simulink model "SecRwRtStBkReclnCtrl"  (R2024b)
settings: Solver=FixedStepDiscrete  StartTime=0.0  StopTime=10.0  FixedStep=0.01  RelTol=1e-3
undefined symbols (not defined in the file or in its folder): KeSMSuMdMotFinshdTm_Val, KeSMSuMdRetryTm1_Val, KeSMSuModeReqDurgTm_Val
libraries: StCtrlLibBkRecln x1
settings Model: Creator=sn2xws  LastModifiedBy=sn55gm
settings SolverCC: AlgebraicLoopSolver=TrustRegion
settings DataIOCC: SaveFormat=StructureWithTime  ReturnWorkspaceOutputs=off
settings OptimizationCC: DefaultParameterBehavior=Inlined  EnhancedBackFolding=on  PassReuseOutputArgsAs=Individual arguments  ZeroExternalMemoryAtStartup=off  ZeroInternalMemoryAtStartup=off  OptimizeBlockOrder=speed  DifferentSizesBufferReuse=on  OptimizationCustomize=off  EfficientTunableParamExpr=on
settings DebuggingCC: ParameterTunabilityLossMsg=error  UnconnectedInputMsg=warning  UnconnectedOutputMsg=warning  UnconnectedLineMsg=warning  ArithmeticOperatorsInVariantConditions=warning
settings ModelReferenceCC: EnableRefExpFcnMdlSchedulingChecks=on  ModelReferenceNumInstancesAllowed=Single
settings SFSimCC: MATLABDynamicMemAlloc=off  CustomCodeUndefinedFunction=UseInterfaceOnly
settings RTWCC: Description=AUTOSAR  SystemTargetFile=autosar.tlc  GenCodeOnly=on  TemplateMakefile=ert_default_tmf  GenerateReport=on  IncludeHyperlinkInReport=on  LaunchReport=on  DataTypeReplacement=CDataTypesFixedWidth  GenerateTraceInfo=on  GenerateTraceReport=on  GenerateTraceReportSl=on  GenerateTraceReportSf=on  GenerateTraceReportEml=on  GPUComputeCapability=3.5
settings CodeAppCC: ForceParamTrailComments=on  IgnoreCustomStorageClasses=off  OperatorAnnotations=on  SimulinkDataObjDesc=on  SFDataObjDesc=on  InsertBlockDesc=on
settings STFCustomTargetCC: TargetLangStandard=C99 (ISO)  MultiwordLength=256  ParMdlRefBuildCompliant=on  CompOptLevelCompliant=on  IncludeMdlTerminateFcn=off  CombineOutputUpdateFcns=on  SuppressErrorStatus=on  ERTCustomFileBanners=on  SupportNonFinite=off  SupportComplex=off  SupportContinuousTime=off  SupportNonInlinedSFcns=off  RemoveResetFunc=on  MATLABClassNameForMDSCustomization=Simulink.SoftwareTarget.ERTCustomization  AutosarCompliant=on  UseToolchainInfoCompliant=on  LookupTableObjectStructAxisOrder=2,1,3,4,...  LUTObjectStructOrderEvenSpacing=Size,Table,Breakpoints  SystemTargetFile=autosar.tlc
settings ERTTargetCC: TargetLangStandard=C99 (ISO)  ConcurrentExecutionCompliant=off  IncludeMdlTerminateFcn=off  SuppressErrorStatus=on  SupportNonFinite=off  SupportComplex=off  ModelStepFunctionPrototypeControlCompliant=off  CPPClassGenCompliant=off  AutosarCompliant=on  LookupTableObjectStructAxisOrder=2,1,3,4,...  LUTObjectStructOrderEvenSpacing=Size,Table,Breakpoints  ERTCustomFileTemplate=example_file_process.tlc  ERTFilePackagingFormat=Compact  BooleanTrueId=TRUE  BooleanFalseId=FALSE  DynamicArrayContainerType=coder::array

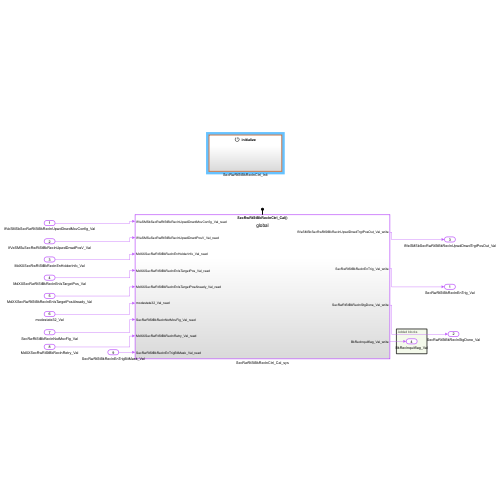
[thumbnail: Simulink's stored preview of the top-level diagram]
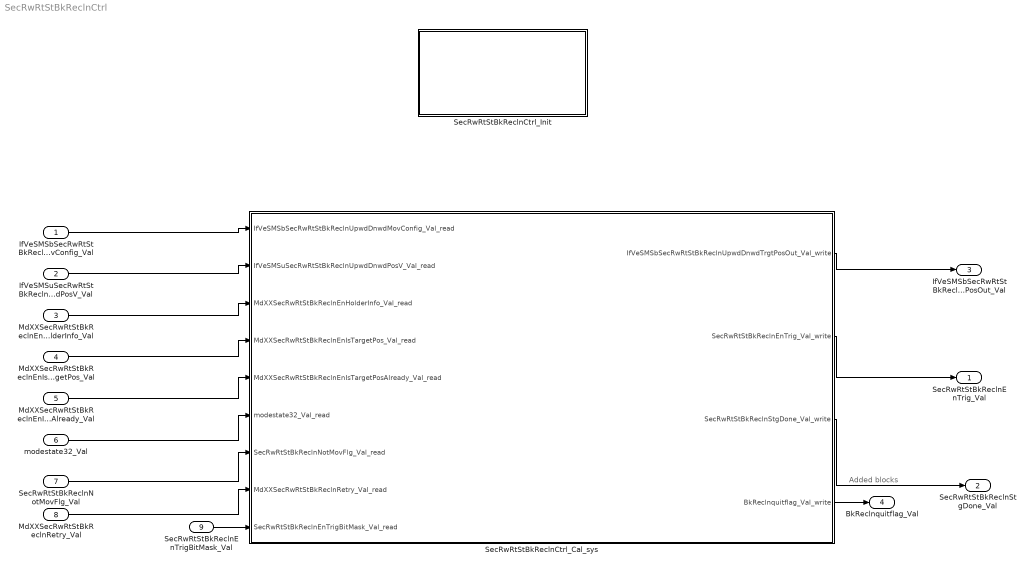
== system SecRwRtStBkReclnCtrl ==
  note: Added blocks
  IfVeSMSbSecRwRtStBkReclnUpwdDnwdMovConfig_Val : Inport  OutDataTypeStr=boolean  PortDimensions=1
  IfVeSMSuSecRwRtStBkReclnUpwdDnwdPosV_Val : Inport  Port=2  OutDataTypeStr=boolean  PortDimensions=1
  MdXXSecRwRtStBkReclnEnHolderInfo_Val : Inport  Port=3  OutDataTypeStr=uint32  PortDimensions=1
  MdXXSecRwRtStBkReclnEnIsTargetPos_Val : Inport  Port=4  OutDataTypeStr=uint32  PortDimensions=1
  MdXXSecRwRtStBkReclnEnIsTargetPosAlready_Val : Inport  Port=5  OutDataTypeStr=uint32  PortDimensions=1
  modestate32_Val : Inport  Port=6  OutDataTypeStr=uint32  PortDimensions=1
  SecRwRtStBkReclnNotMovFlg_Val : Inport  Port=7  OutDataTypeStr=boolean  PortDimensions=1
  MdXXSecRwRtStBkReclnRetry_Val : Inport  Port=8  OutDataTypeStr=uint32  PortDimensions=1
  SecRwRtStBkReclnEnTrigBitMask_Val : Inport  Port=9  OutDataTypeStr=uint32  PortDimensions=1
  SecRwRtStBkReclnCtrl_Cal_sys : Subsystem
  SecRwRtStBkReclnCtrl_Init : Subsystem
  SecRwRtStBkReclnEnTrig_Val : Outport  OutDataTypeStr=boolean  PortDimensions=1  VectorParamsAs1DForOutWhenUnconnected=off
  SecRwRtStBkReclnStgDone_Val : Outport  Port=2  OutDataTypeStr=boolean  PortDimensions=1  VectorParamsAs1DForOutWhenUnconnected=off
  IfVeSMSbSecRwRtStBkReclnUpwdDnwdTrgtPosOut_Val : Outport  Port=3  OutDataTypeStr=boolean  PortDimensions=1  VectorParamsAs1DForOutWhenUnconnected=off
  BkReclnquitflag_Val : Outport  Port=4  OutDataTypeStr=boolean  PortDimensions=1  VectorParamsAs1DForOutWhenUnconnected=off
  wires:
  IfVeSMSbSecRwRtStBkReclnUpwdDnwdMovConfig_Val/1 -> SecRwRtStBkReclnCtrl_Cal_sys/1(IfVeSMSbSecRwRtStBkReclnUpwdDnwdMovConfig_Val_read)
  IfVeSMSuSecRwRtStBkReclnUpwdDnwdPosV_Val/1 -> SecRwRtStBkReclnCtrl_Cal_sys/2(IfVeSMSuSecRwRtStBkReclnUpwdDnwdPosV_Val_read)
  MdXXSecRwRtStBkReclnEnHolderInfo_Val/1 -> SecRwRtStBkReclnCtrl_Cal_sys/3(MdXXSecRwRtStBkReclnEnHolderInfo_Val_read)
  MdXXSecRwRtStBkReclnEnIsTargetPos_Val/1 -> SecRwRtStBkReclnCtrl_Cal_sys/4(MdXXSecRwRtStBkReclnEnIsTargetPos_Val_read)
  MdXXSecRwRtStBkReclnEnIsTargetPosAlready_Val/1 -> SecRwRtStBkReclnCtrl_Cal_sys/5(MdXXSecRwRtStBkReclnEnIsTargetPosAlready_Val_read)
  modestate32_Val/1 -> SecRwRtStBkReclnCtrl_Cal_sys/6(modestate32_Val_read)
  SecRwRtStBkReclnNotMovFlg_Val/1 -> SecRwRtStBkReclnCtrl_Cal_sys/7(SecRwRtStBkReclnNotMovFlg_Val_read)
  SecRwRtStBkReclnCtrl_Cal_sys/1(IfVeSMSbSecRwRtStBkReclnUpwdDnwdTrgtPosOut_Val_write) -> IfVeSMSbSecRwRtStBkReclnUpwdDnwdTrgtPosOut_Val/1
  SecRwRtStBkReclnCtrl_Cal_sys/2(SecRwRtStBkReclnEnTrig_Val_write) -> SecRwRtStBkReclnEnTrig_Val/1
  SecRwRtStBkReclnCtrl_Cal_sys/3(SecRwRtStBkReclnStgDone_Val_write) -> SecRwRtStBkReclnStgDone_Val/1
  MdXXSecRwRtStBkReclnRetry_Val/1 -> SecRwRtStBkReclnCtrl_Cal_sys/8(MdXXSecRwRtStBkReclnRetry_Val_read)
  SecRwRtStBkReclnEnTrigBitMask_Val/1 -> SecRwRtStBkReclnCtrl_Cal_sys/9(SecRwRtStBkReclnEnTrigBitMask_Val_read)
  SecRwRtStBkReclnCtrl_Cal_sys/4(BkReclnquitflag_Val_write) -> BkReclnquitflag_Val/1

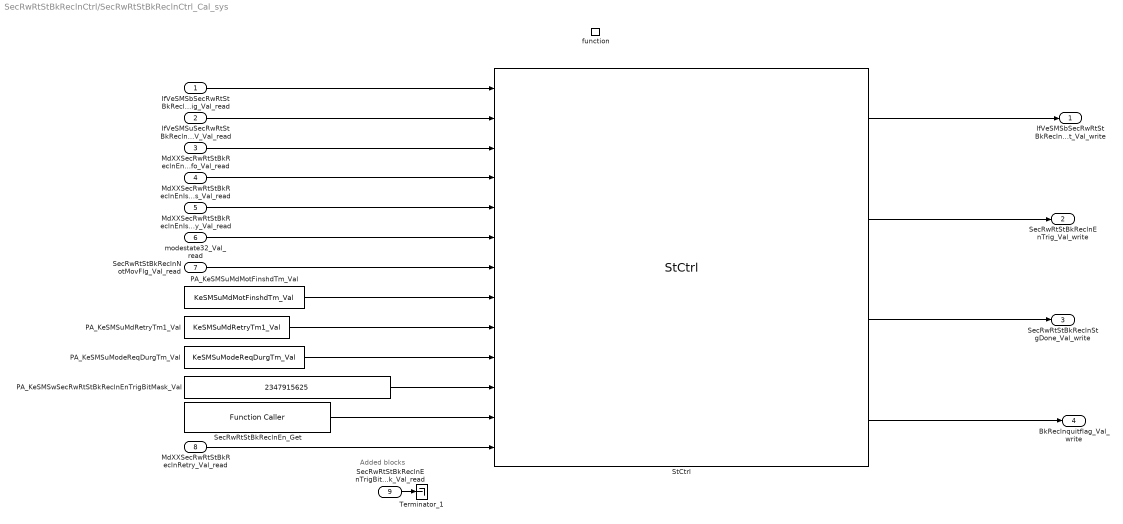
== system SecRwRtStBkReclnCtrl/SecRwRtStBkReclnCtrl_Cal_sys ==
  note: Added blocks
  IfVeSMSbSecRwRtStBkReclnUpwdDnwdMovConfig_Val_read : Inport
  IfVeSMSuSecRwRtStBkReclnUpwdDnwdPosV_Val_read : Inport  Port=2
  MdXXSecRwRtStBkReclnEnHolderInfo_Val_read : Inport  Port=3
  MdXXSecRwRtStBkReclnEnIsTargetPos_Val_read : Inport  Port=4
  MdXXSecRwRtStBkReclnEnIsTargetPosAlready_Val_read : Inport  Port=5
  modestate32_Val_read : Inport  Port=6
  SecRwRtStBkReclnNotMovFlg_Val_read : Inport  Port=7
  MdXXSecRwRtStBkReclnRetry_Val_read : Inport  Port=8
  SecRwRtStBkReclnEnTrigBitMask_Val_read : Inport  Port=9
  function : TriggerPort  TriggerType=function-call  IsSimulinkFunction=on  FunctionName=SecRwRtStBkReclnCtrl_Cal  VariantControl=(inherit)
  PA_KeSMSuMdMotFinshdTm_Val : Constant  Value=KeSMSuMdMotFinshdTm_Val
  PA_KeSMSuMdRetryTm1_Val : Constant  Value=KeSMSuMdRetryTm1_Val
  PA_KeSMSuModeReqDurgTm_Val : Constant  Value=KeSMSuModeReqDurgTm_Val
  PA_KeSMSwSecRwRtStBkReclnEnTrigBitMask_Val : Constant  Value=2347915625  OutDataTypeStr=uint32
  SecRwRtStBkReclnEn_Get : FunctionCaller  FunctionPrototype=data = SecRwRtStBkReclnEn_Get()  InputArgumentSpecifications=<Enter example>  OutputArgumentSpecifications=uint32(1)
  StCtrl : StCtrlLibBkRecln/StCtrl  SystemSampleTime=-1  VariantActivationTime=update diagram  AllowFlexibleInterface=on  Latency=0  AutoFrameSizeCalculation=off
  Terminator_1 : Terminator
  IfVeSMSbSecRwRtStBkReclnUpwdDnwdTrgtPosOut_Val_write : Outport  VectorParamsAs1DForOutWhenUnconnected=off
      settings: EnsureOutportIsVirtual=on
  SecRwRtStBkReclnEnTrig_Val_write : Outport  Port=2  VectorParamsAs1DForOutWhenUnconnected=off
      settings: EnsureOutportIsVirtual=on
  SecRwRtStBkReclnStgDone_Val_write : Outport  Port=3  VectorParamsAs1DForOutWhenUnconnected=off
      settings: EnsureOutportIsVirtual=on
  BkReclnquitflag_Val_write : Outport  Port=4  VectorParamsAs1DForOutWhenUnconnected=off
      settings: EnsureOutportIsVirtual=on
  wires:
  StCtrl/1 -> IfVeSMSbSecRwRtStBkReclnUpwdDnwdTrgtPosOut_Val_write/1
  StCtrl/2 -> SecRwRtStBkReclnEnTrig_Val_write/1
  StCtrl/3 -> SecRwRtStBkReclnStgDone_Val_write/1
  PA_KeSMSwSecRwRtStBkReclnEnTrigBitMask_Val/1 -> StCtrl/11
  SecRwRtStBkReclnEn_Get/1 -> StCtrl/12
  PA_KeSMSuMdMotFinshdTm_Val/1 -> StCtrl/8
  PA_KeSMSuModeReqDurgTm_Val/1 -> StCtrl/10
  PA_KeSMSuMdRetryTm1_Val/1 -> StCtrl/9
  MdXXSecRwRtStBkReclnEnHolderInfo_Val_read/1 -> StCtrl/3
  MdXXSecRwRtStBkReclnEnIsTargetPos_Val_read/1 -> StCtrl/4
  IfVeSMSuSecRwRtStBkReclnUpwdDnwdPosV_Val_read/1 -> StCtrl/2
  MdXXSecRwRtStBkReclnEnIsTargetPosAlready_Val_read/1 -> StCtrl/5
  IfVeSMSbSecRwRtStBkReclnUpwdDnwdMovConfig_Val_read/1 -> StCtrl/1
  modestate32_Val_read/1 -> StCtrl/6
  SecRwRtStBkReclnNotMovFlg_Val_read/1 -> StCtrl/7
  MdXXSecRwRtStBkReclnRetry_Val_read/1 -> StCtrl/13
  SecRwRtStBkReclnEnTrigBitMask_Val_read/1 -> Terminator_1/1
  StCtrl/4 -> BkReclnquitflag_Val_write/1

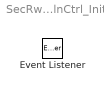
== system SecRwRtStBkReclnCtrl/SecRwRtStBkReclnCtrl_Init ==
  Event Listener : EventListener  EventName=reset
